simulink model "HPC"  (R2025a)
settings: Solver=VariableStepAuto  StartTime=0.0  StopTime=10.0  RelTol=1e-3
undefined symbols (not defined in the file or in its folder): effMod_HPC, eta_hpc_map, PR_hpc_map, speed_vec_hpc, Wc_hpc_bp
settings Model: Creator=ramch  LastModifiedBy=ramch

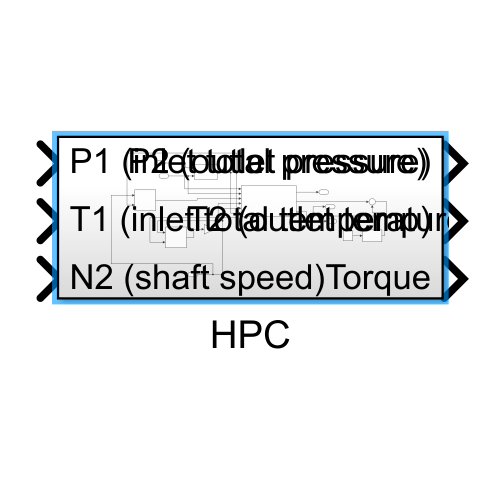
[thumbnail: Simulink's stored preview of the top-level diagram]
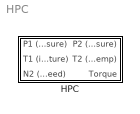
== system HPC ==
  HPC : Subsystem

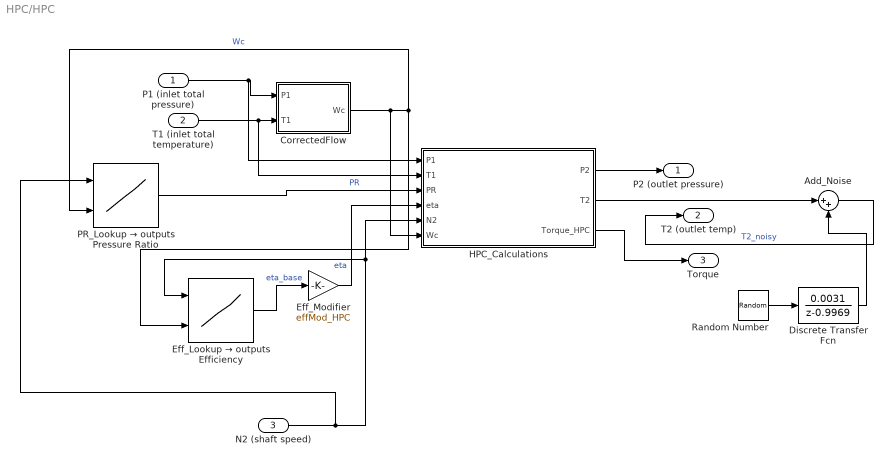
== system HPC/HPC ==
  P1 (inlet total pressure) : Inport
  "T1 (inlet total temperature) " : Inport  Port=2
  N2 (shaft speed) : Inport  Port=3
  Add_Noise : Sum  Inputs=|++
  CorrectedFlow : MATLAB Function  TreatAsAtomicUnit=on
  Discrete Transfer Fcn : DiscreteTransferFcn  Numerator=0.0031  Denominator=1 -0.9969  InitialStates=0.001
  Eff_Lookup → outputs Efficiency : Lookup_n-D  BreakpointsForDimension1=speed_vec_hpc  BreakpointsForDimension2=Wc_hpc_bp  Table=eta_hpc_map  InternalRulePriority=Speed  RndMeth=Simplest
      settings: InputPortMap=u0,u1
  Eff_Modifier : Gain  Gain=effMod_HPC
  HPC_Calculations : MATLAB Function  TreatAsAtomicUnit=on
  PR_Lookup → outputs Pressure Ratio : Lookup_n-D  BreakpointsForDimension1=speed_vec_hpc  BreakpointsForDimension2=Wc_hpc_bp  Table=PR_hpc_map  InternalRulePriority=Speed  RndMeth=Simplest
      settings: InputPortMap=u0,u1
  Random Number : RandomNumber  Variance=(0.5)  SampleTime=0.001
  P2 (outlet pressure) : Outport
  T2 (outlet temp) : Outport  Port=2
  Torque : Outport  Port=3
  wires:
  HPC_Calculations/1(P2) -> P2 (outlet pressure)/1
  HPC_Calculations/2(T2) -> Add_Noise/1
  HPC_Calculations/3(Torque_HPC) -> Torque/1
  PR_Lookup → outputs Pressure Ratio/1 -> HPC_Calculations/3(PR)  "PR"
  Eff_Lookup → outputs Efficiency/1 -> Eff_Modifier/1  "eta_base"
  N2 (shaft speed)/1 -> PR_Lookup → outputs Pressure Ratio/1, Eff_Lookup → outputs Efficiency/1, HPC_Calculations/5(N2)
  P1 (inlet total pressure)/1 -> HPC_Calculations/1(P1), CorrectedFlow/1(P1)
  "T1 (inlet total temperature) "/1 -> HPC_Calculations/2(T1), CorrectedFlow/2(T1)
  CorrectedFlow/1(Wc) -> HPC_Calculations/6(Wc), PR_Lookup → outputs Pressure Ratio/2, Eff_Lookup → outputs Efficiency/2  "Wc"
  Eff_Modifier/1 -> HPC_Calculations/4(eta)  "eta"
  Add_Noise/1 -> T2 (outlet temp)/1  "T2_noisy"
  Discrete Transfer Fcn/1 -> Add_Noise/2
  Random Number/1 -> Discrete Transfer Fcn/1

== matlab function HPC/CorrectedFlow ==
  data: P1 input; Wc output; T1 input
function Wc = Calc_Wc(P1, T1)
% Computes corrected mass flow [kg/s] from inlet P1, T1
    Tref = 288.15;      % Reference temperature [K]
    Pref = 101325;      % Reference pressure [Pa]
    R = 287;            % J/(kg·K), gas constant for air
    A = 0.05;           % Inlet area [m^2] (choose as engine geometry)
    V = 100;            % Inlet velocity [m/s] (estimate)
    % Ideal-gas density at inlet
    rho = P1 / (R * T1);
    % Actual mass flow
    m_dot = rho * A * V;            % [kg/s]
    % Corrected mass flow
    Wc = m_dot / sqrt(T1 / Tref) * (Pref / P1);
end

== matlab function HPC/HPC_Calculations ==
  data: P1 input; P2 output; T1 input; PR input; eta input; N2 input; T2 output; Torque_HPC output; Wc input
function [P2, T2, Torque_HPC] = HPC_CoreCalc(P1, T1, PR, eta, N2, Wc)
% Computes P2, T2, and torque on N2 shaft

    % Constants
    gamma = 1.4;  % Specific heat ratio for air
    cp = 1004;    % J/(kg·K), specific heat at constant pressure
    
    % 1) Outlet total pressure
    P2 = P1 * PR;
    
    % 2) Outlet total temperature (isentropic relation corrected by eta)
    T2 = T1 * (1 + (1/eta) * (PR^((gamma-1)/gamma) - 1));
    
    % 3) Convert shaft speed N2 [RPM] to rad/s
    omega = N2 * 2 * pi / 60;
    
    % 4) Compute actual mass flow from corrected Wc:
    %    Inverse of correction: m_dot = Wc * sqrt(T1/Tref) * (P1/Pref).
    Tref = 288.15;
    Pref = 101325;
    m_dot = Wc * sqrt(T1/Tref) * (P1/Pref);  % [kg/s]
    
    % 5) Compute enthalpy rise Δh = cp*(T2 - T1)
    delta_h = cp * (T2 - T1);  % [J/kg]
    
    % 6) Torque on shaft: (ṁ * Δh) / ω
    Torque_HPC = (m_dot * delta_h) / omega;  % [N·m]
end
